simulink model "Stabilize_mode_discretized"  (R2016a)
settings: Solver=VariableStepAuto  StartTime=0.0  StopTime=10  FixedStep=0.0000001  RelTol=1e-3
model workspace (MAT data in the model file):
  AC_ATTITUDE_ACCEL_Y_CONTROLLER_MAX_RADSS = Simulink.Signal
  AC_ATTITUDE_ACCEL_Y_CONTROLLER_MAX_RADSS.DataType = 'double'
  AC_ATTITUDE_ACCEL_Y_CONTROLLER_MAX_RADSS.Dimensions = 1
  AC_ATTITUDE_ACCEL_Y_CONTROLLER_MAX_RADSS.DimensionsMode = 'auto'
  AC_ATTITUDE_ACCEL_Y_CONTROLLER_MAX_RADSS.Complexity = 'real'
  AC_ATTITUDE_ACCEL_Y_CONTROLLER_MAX_RADSS.SampleTime = -1
  AC_ATTITUDE_ACCEL_Y_CONTROLLER_MAX_RADSS.SamplingMode = 'Sample based'
  AC_ATTITUDE_ACCEL_Y_CONTROLLER_MAX_RADSS.InitialValue = '0.5'
  AC_ATTITUDE_CONTROL_MAX = Simulink.Signal
  AC_ATTITUDE_CONTROL_MAX.DataType = 'double'
  AC_ATTITUDE_CONTROL_MAX.Dimensions = 1
  AC_ATTITUDE_CONTROL_MAX.DimensionsMode = 'auto'
  AC_ATTITUDE_CONTROL_MAX.Complexity = 'real'
  AC_ATTITUDE_CONTROL_MAX.SampleTime = -1
  AC_ATTITUDE_CONTROL_MAX.SamplingMode = 'Sample based'
  AC_ATTITUDE_CONTROL_MAX.InitialValue = '0.5'
  AC_ATTITUDE_THRUST_ERROR_ANGLE = Simulink.Signal
  AC_ATTITUDE_THRUST_ERROR_ANGLE.DataType = 'double'
  AC_ATTITUDE_THRUST_ERROR_ANGLE.Dimensions = 1
  AC_ATTITUDE_THRUST_ERROR_ANGLE.DimensionsMode = 'auto'
  AC_ATTITUDE_THRUST_ERROR_ANGLE.Complexity = 'real'
  AC_ATTITUDE_THRUST_ERROR_ANGLE.SampleTime = -1
  AC_ATTITUDE_THRUST_ERROR_ANGLE.SamplingMode = 'Sample based'
  AC_ATTITUDE_THRUST_ERROR_ANGLE.InitialValue = '1000'
  ROLL_PITCH_INPUT_MAX = Simulink.Signal
  ROLL_PITCH_INPUT_MAX.DataType = 'double'
  ROLL_PITCH_INPUT_MAX.Dimensions = 1
  ROLL_PITCH_INPUT_MAX.DimensionsMode = 'auto'
  ROLL_PITCH_INPUT_MAX.Complexity = 'real'
  ROLL_PITCH_INPUT_MAX.SampleTime = -1
  ROLL_PITCH_INPUT_MAX.SamplingMode = 'Sample based'
  ROLL_PITCH_INPUT_MAX.InitialValue = '3000'
  Sig = Simulink.Signal
  Sig.DataType = 'auto'
  Sig.Dimensions = -1
  Sig.DimensionsMode = 'auto'
  Sig.Complexity = 'auto'
  Sig.SampleTime = -1
  Sig.SamplingMode = 'auto'
  Sig1 = Simulink.Signal
  Sig1.DataType = 'auto'
  Sig1.Dimensions = -1
  Sig1.DimensionsMode = 'auto'
  Sig1.Complexity = 'auto'
  Sig1.SampleTime = -1
  Sig1.SamplingMode = 'auto'
  acro_yaw_p = Simulink.Signal
  acro_yaw_p.DataType = 'double'
  acro_yaw_p.Dimensions = 1
  acro_yaw_p.DimensionsMode = 'auto'
  acro_yaw_p.Complexity = 'real'
  acro_yaw_p.SampleTime = -1
  acro_yaw_p.SamplingMode = 'Sample based'
  acro_yaw_p.InitialValue = '45'
  angle_max = Simulink.Signal
  angle_max.DataType = 'double'
  angle_max.Dimensions = 1
  angle_max.DimensionsMode = 'auto'
  angle_max.Complexity = 'real'
  angle_max.SampleTime = -1
  angle_max.SamplingMode = 'Sample based'
  angle_max.InitialValue = '3000'
  attitude_target_ang_vel = Simulink.Signal
  attitude_target_ang_vel.DataType = 'double'
  attitude_target_ang_vel.Dimensions = 3
  attitude_target_ang_vel.DimensionsMode = 'auto'
  attitude_target_ang_vel.Complexity = 'real'
  attitude_target_ang_vel.SampleTime = -1
  attitude_target_ang_vel.SamplingMode = 'Sample based'
  attitude_target_ang_vel.InitialValue = '[0 0 0]'
  attitude_target_euler_angle_x = Simulink.Signal
  attitude_target_euler_angle_x.DataType = 'double'
  attitude_target_euler_angle_x.Dimensions = 1
  attitude_target_euler_angle_x.DimensionsMode = 'auto'
  attitude_target_euler_angle_x.Complexity = 'real'
  attitude_target_euler_angle_x.SampleTime = -1
  attitude_target_euler_angle_x.SamplingMode = 'Sample based'
  attitude_target_euler_angle_x.InitialValue = '0'
  attitude_target_euler_angle_y = Simulink.Signal
  attitude_target_euler_angle_y.DataType = 'double'
  attitude_target_euler_angle_y.Dimensions = 1
  attitude_target_euler_angle_y.DimensionsMode = 'auto'
  attitude_target_euler_angle_y.Complexity = 'real'
  attitude_target_euler_angle_y.SampleTime = -1
  attitude_target_euler_angle_y.SamplingMode = 'Sample based'
  attitude_target_euler_angle_y.InitialValue = '0'
  attitude_target_euler_angle_z = Simulink.Signal
  attitude_target_euler_angle_z.DataType = 'double'
  attitude_target_euler_angle_z.Dimensions = 1
  attitude_target_euler_angle_z.DimensionsMode = 'auto'
  attitude_target_euler_angle_z.Complexity = 'real'
  attitude_target_euler_angle_z.SampleTime = -1
  attitude_target_euler_angle_z.SamplingMode = 'Sample based'
  attitude_target_euler_angle_z.InitialValue = '0'
  attitude_target_euler_rate = Simulink.Signal
  attitude_target_euler_rate.DataType = 'double'
  attitude_target_euler_rate.Dimensions = 3
  attitude_target_euler_rate.DimensionsMode = 'auto'
  attitude_target_euler_rate.Complexity = 'real'
  attitude_target_euler_rate.SampleTime = -1
  attitude_target_euler_rate.SamplingMode = 'Sample based'
  attitude_target_euler_rate.InitialValue = '[0 0 0]'
  attitude_target_quat = Simulink.Signal
  attitude_target_quat.DataType = 'double'
  attitude_target_quat.Dimensions = 4
  attitude_target_quat.DimensionsMode = 'auto'
  attitude_target_quat.Complexity = 'real'
  attitude_target_quat.SampleTime = -1
  attitude_target_quat.SamplingMode = 'Sample based'
  attitude_target_quat.InitialValue = '[1 0 0 0]'
  attitude_vehicle_quat = Simulink.Signal
  attitude_vehicle_quat.DataType = 'double'
  attitude_vehicle_quat.Dimensions = 4
  attitude_vehicle_quat.DimensionsMode = 'auto'
  attitude_vehicle_quat.Complexity = 'real'
  attitude_vehicle_quat.SampleTime = -1
  attitude_vehicle_quat.SamplingMode = 'Sample based'
  attitude_vehicle_quat.InitialValue = '[1 0 0 0]'
  dt = Simulink.Signal
  dt.DataType = 'double'
  dt.Dimensions = 1
  dt.DimensionsMode = 'auto'
  dt.Complexity = 'real'
  dt.SampleTime = -1
  dt.SamplingMode = 'Sample based'
  dt.InitialValue = '0.01'
  false = 0
  limit_roll_pitch = Simulink.Signal
  limit_roll_pitch.DataType = 'double'
  limit_roll_pitch.Dimensions = 1
  limit_roll_pitch.DimensionsMode = 'auto'
  limit_roll_pitch.Complexity = 'real'
  limit_roll_pitch.SampleTime = -1
  limit_roll_pitch.SamplingMode = 'Sample based'
  limit_roll_pitch.InitialValue = '0.0'
  limit_throttle_upper = Simulink.Signal
  limit_throttle_upper.DataType = 'logical'
  limit_throttle_upper.Dimensions = 1
  limit_throttle_upper.DimensionsMode = 'auto'
  limit_throttle_upper.Complexity = 'real'
  limit_throttle_upper.SampleTime = -1
  limit_throttle_upper.SamplingMode = 'Sample based'
  limit_throttle_upper.InitialValue = '0'
  limit_yaw = Simulink.Signal
  limit_yaw.DataType = 'double'
  limit_yaw.Dimensions = 1
  limit_yaw.DimensionsMode = 'auto'
  limit_yaw.Complexity = 'real'
  limit_yaw.SampleTime = -1
  limit_yaw.SamplingMode = 'Sample based'
  limit_yaw.InitialValue = '0'
  loop_rate = Simulink.Signal
  loop_rate.DataType = 'double'
  loop_rate.Dimensions = 1
  loop_rate.DimensionsMode = 'auto'
  loop_rate.Complexity = 'real'
  loop_rate.SampleTime = -1
  loop_rate.SamplingMode = 'Sample based'
  loop_rate.InitialValue = '100'
  pitch_attitude_kP = Simulink.Signal
  pitch_attitude_kP.DataType = 'double'
  pitch_attitude_kP.Dimensions = 1
  pitch_attitude_kP.DimensionsMode = 'auto'
  pitch_attitude_kP.Complexity = 'real'
  pitch_attitude_kP.SampleTime = -1
  pitch_attitude_kP.SamplingMode = 'Sample based'
  pitch_attitude_kP.InitialValue = '20'
  pitch_factor = Simulink.Signal
  pitch_factor.DataType = 'double'
  pitch_factor.Dimensions = 4
  pitch_factor.DimensionsMode = 'auto'
  pitch_factor.Complexity = 'real'
  pitch_factor.SampleTime = -1
  pitch_factor.SamplingMode = 'Sample based'
  pitch_factor.InitialValue = '[cos(deg2rad(15)) -cos(deg2rad(15)) cos(deg2rad(15)) -cos(deg2rad(15))]'
  pitch_rate_derivative = Simulink.Signal
  pitch_rate_derivative.DataType = 'double'
  pitch_rate_derivative.Dimensions = 1
  pitch_rate_derivative.DimensionsMode = 'auto'
  pitch_rate_derivative.Complexity = 'real'
  pitch_rate_derivative.SampleTime = -1
  pitch_rate_derivative.SamplingMode = 'Sample based'
  pitch_rate_derivative.InitialValue = '0'
  pitch_rate_error_rads = Simulink.Signal
  pitch_rate_error_rads.DataType = 'double'
  pitch_rate_error_rads.Dimensions = 1
  pitch_rate_error_rads.DimensionsMode = 'auto'
  pitch_rate_error_rads.Complexity = 'real'
  pitch_rate_error_rads.SampleTime = -1
  pitch_rate_error_rads.SamplingMode = 'Sample based'
  pitch_rate_error_rads.InitialValue = '0'
  pitch_rate_filt_hz = Simulink.Signal
  pitch_rate_filt_hz.DataType = 'double'
  pitch_rate_filt_hz.Dimensions = 1
  pitch_rate_filt_hz.DimensionsMode = 'auto'
  pitch_rate_filt_hz.Complexity = 'real'
  pitch_rate_filt_hz.SampleTime = -1
  pitch_rate_filt_hz.SamplingMode = 'Sample based'
  pitch_rate_filt_hz.InitialValue = '1/(2*pi)'
  pitch_rate_imax = Simulink.Signal
  pitch_rate_imax.DataType = 'double'
  pitch_rate_imax.Dimensions = 1
  pitch_rate_imax.DimensionsMode = 'auto'
  pitch_rate_imax.Complexity = 'real'
  pitch_rate_imax.SampleTime = -1
  pitch_rate_imax.SamplingMode = 'Sample based'
  pitch_rate_imax.InitialValue = '200'
  pitch_rate_integrator = Simulink.Signal
  pitch_rate_integrator.DataType = 'double'
  pitch_rate_integrator.Dimensions = 1
  pitch_rate_integrator.DimensionsMode = 'auto'
  pitch_rate_integrator.Complexity = 'real'
  pitch_rate_integrator.SampleTime = -1
  pitch_rate_integrator.SamplingMode = 'Sample based'
  pitch_rate_integrator.InitialValue = '0'
  pitch_rate_kD = Simulink.Signal
  pitch_rate_kD.DataType = 'double'
  pitch_rate_kD.Dimensions = 1
  pitch_rate_kD.DimensionsMode = 'auto'
  pitch_rate_kD.Complexity = 'real'
  pitch_rate_kD.SampleTime = -1
  pitch_rate_kD.SamplingMode = 'Sample based'
  pitch_rate_kD.InitialValue = '0.004'
  pitch_rate_kI = Simulink.Signal
  pitch_rate_kI.DataType = 'double'
  pitch_rate_kI.Dimensions = 1
  pitch_rate_kI.DimensionsMode = 'auto'
  pitch_rate_kI.Complexity = 'real'
  pitch_rate_kI.SampleTime = -1
  pitch_rate_kI.SamplingMode = 'Sample based'
  pitch_rate_kI.InitialValue = '0.1'
  pitch_rate_kP = Simulink.Signal
  pitch_rate_kP.DataType = 'double'
  pitch_rate_kP.Dimensions = 1
  pitch_rate_kP.DimensionsMode = 'auto'
  pitch_rate_kP.Complexity = 'real'
  pitch_rate_kP.SampleTime = -1
  pitch_rate_kP.SamplingMode = 'Sample based'
  pitch_rate_kP.InitialValue = '0.5'
  pitch_rate_last_input = Simulink.Signal
  pitch_rate_last_input.DataType = 'double'
  pitch_rate_last_input.Dimensions = 1
  pitch_rate_last_input.DimensionsMode = 'auto'
  pitch_rate_last_input.Complexity = 'real'
  pitch_rate_last_input.SampleTime = -1
  pitch_rate_last_input.SamplingMode = 'Sample based'
  pitch_rate_last_input.InitialValue = '0'
  pitch_rate_proportional = Simulink.Signal
  pitch_rate_proportional.DataType = 'double'
  pitch_rate_proportional.Dimensions = 1
  pitch_rate_proportional.DimensionsMode = 'auto'
  pitch_rate_proportional.Complexity = 'real'
  pitch_rate_proportional.SampleTime = -1
  pitch_rate_proportional.SamplingMode = 'Sample based'
  pitch_rate_proportional.InitialValue = '0'
  pwm_max = Simulink.Signal
  pwm_max.DataType = 'double'
  pwm_max.Dimensions = 1
  pwm_max.DimensionsMode = 'auto'
  pwm_max.Complexity = 'real'
  pwm_max.SampleTime = -1
  pwm_max.SamplingMode = 'Sample based'
  pwm_max.InitialValue = '2000'
  pwm_min = Simulink.Signal
  pwm_min.DataType = 'double'
  pwm_min.Dimensions = 1
  pwm_min.DimensionsMode = 'auto'
  pwm_min.Complexity = 'real'
  pwm_min.SampleTime = -1
  pwm_min.SamplingMode = 'Sample based'
  pwm_min.InitialValue = '1039'
  rate_bf_ff_enabled = Simulink.Signal
  rate_bf_ff_enabled.DataType = 'double'
  rate_bf_ff_enabled.Dimensions = 1
  rate_bf_ff_enabled.DimensionsMode = 'auto'
  rate_bf_ff_enabled.Complexity = 'real'
  rate_bf_ff_enabled.SampleTime = -1
  rate_bf_ff_enabled.SamplingMode = 'Sample based'
  rate_bf_ff_enabled.InitialValue = '0'
  rate_target_ang_vel = Simulink.Signal
  rate_target_ang_vel.DataType = 'double'
  rate_target_ang_vel.Dimensions = 3
  rate_target_ang_vel.DimensionsMode = 'auto'
  rate_target_ang_vel.Complexity = 'real'
  rate_target_ang_vel.SampleTime = -1
  rate_target_ang_vel.SamplingMode = 'Sample based'
  rate_target_ang_vel.InitialValue = '[0 0 0]'
  roll_attitude_kP = Simulink.Signal
  roll_attitude_kP.DataType = 'double'
  roll_attitude_kP.Dimensions = 1
  roll_attitude_kP.DimensionsMode = 'auto'
  roll_attitude_kP.Complexity = 'real'
  roll_attitude_kP.SampleTime = -1
  roll_attitude_kP.SamplingMode = 'Sample based'
  roll_attitude_kP.InitialValue = '20'
  roll_factor = Simulink.Signal
  roll_factor.DataType = 'double'
  roll_factor.Dimensions = 4
  roll_factor.DimensionsMode = 'auto'
  roll_factor.Complexity = 'real'
  roll_factor.SampleTime = -1
  roll_factor.SamplingMode = 'Sample based'
  roll_factor.InitialValue = '[-sin(deg2rad(15)) sin(deg2rad(15)) sin(deg2rad(15)) -sin(deg2rad(15))]'
  roll_rate_derivative = Simulink.Signal
  roll_rate_derivative.DataType = 'double'
  roll_rate_derivative.Dimensions = 1
  roll_rate_derivative.DimensionsMode = 'auto'
  roll_rate_derivative.Complexity = 'real'
  roll_rate_derivative.SampleTime = -1
  roll_rate_derivative.SamplingMode = 'Sample based'
  roll_rate_derivative.InitialValue = '0'
  roll_rate_error_rads = Simulink.Signal
  roll_rate_error_rads.DataType = 'double'
  roll_rate_error_rads.Dimensions = 1
  roll_rate_error_rads.DimensionsMode = 'auto'
  roll_rate_error_rads.Complexity = 'real'
  roll_rate_error_rads.SampleTime = -1
  roll_rate_error_rads.SamplingMode = 'Sample based'
  roll_rate_error_rads.InitialValue = '0'
  roll_rate_filt_hz = Simulink.Signal
  roll_rate_filt_hz.DataType = 'double'
  roll_rate_filt_hz.Dimensions = 1
  roll_rate_filt_hz.DimensionsMode = 'auto'
  roll_rate_filt_hz.Complexity = 'real'
  roll_rate_filt_hz.SampleTime = -1
  roll_rate_filt_hz.SamplingMode = 'Sample based'
  roll_rate_filt_hz.InitialValue = '1/(2*pi)'
  roll_rate_imax = Simulink.Signal
  roll_rate_imax.DataType = 'double'
  roll_rate_imax.Dimensions = 1
  roll_rate_imax.DimensionsMode = 'auto'
  roll_rate_imax.Complexity = 'real'
  roll_rate_imax.SampleTime = -1
  roll_rate_imax.SamplingMode = 'Sample based'
  roll_rate_imax.InitialValue = '200'
  roll_rate_integrator = Simulink.Signal
  roll_rate_integrator.DataType = 'double'
  roll_rate_integrator.Dimensions = 1
  roll_rate_integrator.DimensionsMode = 'auto'
  roll_rate_integrator.Complexity = 'real'
  roll_rate_integrator.SampleTime = -1
  roll_rate_integrator.SamplingMode = 'Sample based'
  roll_rate_integrator.InitialValue = '0'
  roll_rate_kD = Simulink.Signal
  roll_rate_kD.DataType = 'double'
  roll_rate_kD.Dimensions = 1
  roll_rate_kD.DimensionsMode = 'auto'
  roll_rate_kD.Complexity = 'real'
  roll_rate_kD.SampleTime = -1
  roll_rate_kD.SamplingMode = 'Sample based'
  roll_rate_kD.InitialValue = '0.004'
  roll_rate_kI = Simulink.Signal
  roll_rate_kI.DataType = 'double'
  roll_rate_kI.Dimensions = 1
  roll_rate_kI.DimensionsMode = 'auto'
  roll_rate_kI.Complexity = 'real'
  roll_rate_kI.SampleTime = -1
  roll_rate_kI.SamplingMode = 'Sample based'
  roll_rate_kI.InitialValue = '0.1'
  roll_rate_kP = Simulink.Signal
  roll_rate_kP.DataType = 'double'
  roll_rate_kP.Dimensions = 1
  roll_rate_kP.DimensionsMode = 'auto'
  roll_rate_kP.Complexity = 'real'
  roll_rate_kP.SampleTime = -1
  roll_rate_kP.SamplingMode = 'Sample based'
  roll_rate_kP.InitialValue = '1'
  roll_rate_last_input = Simulink.Signal
  roll_rate_last_input.DataType = 'double'
  roll_rate_last_input.Dimensions = 1
  roll_rate_last_input.DimensionsMode = 'auto'
  roll_rate_last_input.Complexity = 'real'
  roll_rate_last_input.SampleTime = -1
  roll_rate_last_input.SamplingMode = 'Sample based'
  roll_rate_last_input.InitialValue = '0'
  roll_rate_proportional = Simulink.Signal
  roll_rate_proportional.DataType = 'double'
  roll_rate_proportional.Dimensions = 1
  roll_rate_proportional.DimensionsMode = 'auto'
  roll_rate_proportional.Complexity = 'real'
  roll_rate_proportional.SampleTime = -1
  roll_rate_proportional.SamplingMode = 'Sample based'
  roll_rate_proportional.InitialValue = '0'
  spin_max = Simulink.Signal
  spin_max.DataType = 'double'
  spin_max.Dimensions = 1
  spin_max.DimensionsMode = 'auto'
  spin_max.Complexity = 'real'
  spin_max.SampleTime = -1
  spin_max.SamplingMode = 'Sample based'
  spin_max.InitialValue = '0.95'
  spin_min = Simulink.Signal
  spin_min.DataType = 'double'
  spin_min.Dimensions = 1
  spin_min.DimensionsMode = 'auto'
  spin_min.Complexity = 'real'
  spin_min.SampleTime = -1
  spin_min.SamplingMode = 'Sample based'
  spin_min.InitialValue = '0.15'
  throttle_avg_max = Simulink.Signal
  throttle_avg_max.DataType = 'double'
  throttle_avg_max.Dimensions = 1
  throttle_avg_max.DimensionsMode = 'auto'
  throttle_avg_max.Complexity = 'real'
  throttle_avg_max.SampleTime = -1
  throttle_avg_max.SamplingMode = 'Sample based'
  throttle_avg_max.InitialValue = '0'
  throttle_filter_cutoff_freq = Simulink.Signal
  throttle_filter_cutoff_freq.DataType = 'double'
  throttle_filter_cutoff_freq.Dimensions = 1
  throttle_filter_cutoff_freq.DimensionsMode = 'auto'
  throttle_filter_cutoff_freq.Complexity = 'real'
  throttle_filter_cutoff_freq.SampleTime = -1
  throttle_filter_cutoff_freq.SamplingMode = 'Sample based'
  throttle_filter_cutoff_freq.InitialValue = '0.5'
  throttle_filter_output = Simulink.Signal
  throttle_filter_output.DataType = 'double'
  throttle_filter_output.Dimensions = 1
  throttle_filter_output.DimensionsMode = 'auto'
  throttle_filter_output.Complexity = 'real'
  throttle_filter_output.SampleTime = -1
  throttle_filter_output.SamplingMode = 'Sample based'
  throttle_filter_output.InitialValue = '0'
  throttle_in = Simulink.Signal
  throttle_in.DataType = 'double'
  throttle_in.Dimensions = 1
  throttle_in.DimensionsMode = 'auto'
  throttle_in.Complexity = 'real'
  throttle_in.SampleTime = -1
  throttle_in.SamplingMode = 'Sample based'
  throttle_in.InitialValue = '0'
  throttle_rpy_mix = Simulink.Signal
  throttle_rpy_mix.DataType = 'double'
  throttle_rpy_mix.Dimensions = 1
  throttle_rpy_mix.DimensionsMode = 'auto'
  throttle_rpy_mix.Complexity = 'real'
  throttle_rpy_mix.SampleTime = -1
  throttle_rpy_mix.SamplingMode = 'Sample based'
  throttle_rpy_mix.InitialValue = '0'
  throttle_rpy_mix_desired = Simulink.Signal
  throttle_rpy_mix_desired.DataType = 'double'
  throttle_rpy_mix_desired.Dimensions = 1
  throttle_rpy_mix_desired.DimensionsMode = 'auto'
  throttle_rpy_mix_desired.Complexity = 'real'
  throttle_rpy_mix_desired.SampleTime = -1
  throttle_rpy_mix_desired.SamplingMode = 'Sample based'
  throttle_rpy_mix_desired.InitialValue = '0'
  throttle_thrust = Simulink.Signal
  throttle_thrust.DataType = 'double'
  throttle_thrust.Dimensions = 1
  throttle_thrust.DimensionsMode = 'auto'
  throttle_thrust.Complexity = 'real'
  throttle_thrust.SampleTime = -1
  throttle_thrust.SamplingMode = 'Sample based'
  throttle_thrust.InitialValue = '0'
  throttle_thrust_best_rpy = Simulink.Signal
  throttle_thrust_best_rpy.DataType = 'double'
  throttle_thrust_best_rpy.Dimensions = 1
  throttle_thrust_best_rpy.DimensionsMode = 'auto'
  throttle_thrust_best_rpy.Complexity = 'real'
  throttle_thrust_best_rpy.SampleTime = -1
  throttle_thrust_best_rpy.SamplingMode = 'Sample based'
  throttle_thrust_best_rpy.InitialValue = '0'
  throttle_thrust_max = Simulink.Signal
  throttle_thrust_max.DataType = 'double'
  throttle_thrust_max.Dimensions = 1
  throttle_thrust_max.DimensionsMode = 'auto'
  throttle_thrust_max.Complexity = 'real'
  throttle_thrust_max.SampleTime = -1
  throttle_thrust_max.SamplingMode = 'Sample based'
  throttle_thrust_max.InitialValue = '1'
  thrust_error_angle = Simulink.Signal
  thrust_error_angle.DataType = 'double'
  thrust_error_angle.Dimensions = 1
  thrust_error_angle.DimensionsMode = 'auto'
  thrust_error_angle.Complexity = 'real'
  thrust_error_angle.SampleTime = -1
  thrust_error_angle.SamplingMode = 'Sample based'
  thrust_error_angle.InitialValue = '0'
  thrust_rpyt_out = Simulink.Signal
  thrust_rpyt_out.DataType = 'double'
  thrust_rpyt_out.Dimensions = 4
  thrust_rpyt_out.DimensionsMode = 'auto'
  thrust_rpyt_out.Complexity = 'real'
  thrust_rpyt_out.SampleTime = -1
  thrust_rpyt_out.SamplingMode = 'Sample based'
  thrust_rpyt_out.InitialValue = '[0 0 0 0]'
  true = 1
  use_ff_and_input_shaping = Simulink.Signal
  use_ff_and_input_shaping.DataType = 'double'
  use_ff_and_input_shaping.Dimensions = 1
  use_ff_and_input_shaping.DimensionsMode = 'auto'
  use_ff_and_input_shaping.Complexity = 'real'
  use_ff_and_input_shaping.SampleTime = -1
  use_ff_and_input_shaping.SamplingMode = 'Sample based'
  use_ff_and_input_shaping.InitialValue = '0'
  variableType = 'S'
  yaw_allowed = Simulink.Signal
  yaw_allowed.DataType = 'double'
  yaw_allowed.Dimensions = 1
  yaw_allowed.DimensionsMode = 'auto'
  yaw_allowed.Complexity = 'real'
  yaw_allowed.SampleTime = -1
  yaw_allowed.SamplingMode = 'Sample based'
  yaw_allowed.InitialValue = '1'
  yaw_attitude_kP = Simulink.Signal
  yaw_attitude_kP.DataType = 'double'
  yaw_attitude_kP.Dimensions = 1
  yaw_attitude_kP.DimensionsMode = 'auto'
  yaw_attitude_kP.Complexity = 'real'
  yaw_attitude_kP.SampleTime = -1
  yaw_attitude_kP.SamplingMode = 'Sample based'
  yaw_attitude_kP.InitialValue = '4.5'
  yaw_factor = Simulink.Signal
  yaw_factor.DataType = 'double'
  yaw_factor.Dimensions = 4
  yaw_factor.DimensionsMode = 'auto'
  yaw_factor.Complexity = 'real'
  yaw_factor.SampleTime = -1
  yaw_factor.SamplingMode = 'Sample based'
  yaw_factor.InitialValue = '[0.1 0.1 -0.1 -0.1]'
  yaw_headroom = Simulink.Signal
  yaw_headroom.DataType = 'double'
  yaw_headroom.Dimensions = 1
  yaw_headroom.DimensionsMode = 'auto'
  yaw_headroom.Complexity = 'real'
  yaw_headroom.SampleTime = -1
  yaw_headroom.SamplingMode = 'Sample based'
  yaw_headroom.InitialValue = '200'
  yaw_rate_derivative = Simulink.Signal
  yaw_rate_derivative.DataType = 'double'
  yaw_rate_derivative.Dimensions = 1
  yaw_rate_derivative.DimensionsMode = 'auto'
  yaw_rate_derivative.Complexity = 'real'
  yaw_rate_derivative.SampleTime = -1
  yaw_rate_derivative.SamplingMode = 'Sample based'
  yaw_rate_derivative.InitialValue = '0'
  yaw_rate_error_rads = Simulink.Signal
  yaw_rate_error_rads.DataType = 'double'
  yaw_rate_error_rads.Dimensions = 1
  yaw_rate_error_rads.DimensionsMode = 'auto'
  yaw_rate_error_rads.Complexity = 'real'
  yaw_rate_error_rads.SampleTime = -1
  yaw_rate_error_rads.SamplingMode = 'Sample based'
  yaw_rate_error_rads.InitialValue = '0'
  yaw_rate_filt_hz = Simulink.Signal
  yaw_rate_filt_hz.DataType = 'double'
  yaw_rate_filt_hz.Dimensions = 1
  yaw_rate_filt_hz.DimensionsMode = 'auto'
  yaw_rate_filt_hz.Complexity = 'real'
  yaw_rate_filt_hz.SampleTime = -1
  yaw_rate_filt_hz.SamplingMode = 'Sample based'
  yaw_rate_filt_hz.InitialValue = '1/(2*pi)'
  yaw_rate_imax = Simulink.Signal
  yaw_rate_imax.DataType = 'double'
  yaw_rate_imax.Dimensions = 1
  yaw_rate_imax.DimensionsMode = 'auto'
  yaw_rate_imax.Complexity = 'real'
  yaw_rate_imax.SampleTime = -1
  yaw_rate_imax.SamplingMode = 'Sample based'
  yaw_rate_imax.InitialValue = '200'
  yaw_rate_integrator = Simulink.Signal
  yaw_rate_integrator.DataType = 'double'
  yaw_rate_integrator.Dimensions = 1
  yaw_rate_integrator.DimensionsMode = 'auto'
  yaw_rate_integrator.Complexity = 'real'
  yaw_rate_integrator.SampleTime = -1
  yaw_rate_integrator.SamplingMode = 'Sample based'
  yaw_rate_integrator.InitialValue = '0'
  yaw_rate_kD = Simulink.Signal
  yaw_rate_kD.DataType = 'double'
  yaw_rate_kD.Dimensions = 1
  yaw_rate_kD.DimensionsMode = 'auto'
  yaw_rate_kD.Complexity = 'real'
  yaw_rate_kD.SampleTime = -1
  yaw_rate_kD.SamplingMode = 'Sample based'
  yaw_rate_kD.InitialValue = '5'
  yaw_rate_kI = Simulink.Signal
  yaw_rate_kI.DataType = 'double'
  yaw_rate_kI.Dimensions = 1
  yaw_rate_kI.DimensionsMode = 'auto'
  yaw_rate_kI.Complexity = 'real'
  yaw_rate_kI.SampleTime = -1
  yaw_rate_kI.SamplingMode = 'Sample based'
  yaw_rate_kI.InitialValue = '0.1'
  yaw_rate_kP = Simulink.Signal
  yaw_rate_kP.DataType = 'double'
  yaw_rate_kP.Dimensions = 1
  yaw_rate_kP.DimensionsMode = 'auto'
  yaw_rate_kP.Complexity = 'real'
  yaw_rate_kP.SampleTime = -1
  yaw_rate_kP.SamplingMode = 'Sample based'
  yaw_rate_kP.InitialValue = '0.2'
  yaw_rate_last_input = Simulink.Signal
  yaw_rate_last_input.DataType = 'double'
  yaw_rate_last_input.Dimensions = 1
  yaw_rate_last_input.DimensionsMode = 'auto'
  yaw_rate_last_input.Complexity = 'real'
  yaw_rate_last_input.SampleTime = -1
  yaw_rate_last_input.SamplingMode = 'Sample based'
  yaw_rate_last_input.InitialValue = '0'
  yaw_rate_proportional = Simulink.Signal
  yaw_rate_proportional.DataType = 'double'
  yaw_rate_proportional.Dimensions = 1
  yaw_rate_proportional.DimensionsMode = 'auto'
  yaw_rate_proportional.Complexity = 'real'
  yaw_rate_proportional.SampleTime = -1
  yaw_rate_proportional.SamplingMode = 'Sample based'
  yaw_rate_proportional.InitialValue = '0'
values from neighbouring files (symbols this model uses):
  A = [0 0  0 1 0 0 0 0 0 0 0 0 ... (first row only)    [attitudeMatrices.m]
  B = [0   0   0    0    0    0 ... (first row only)    [attitudeMatrices.m]
  C = [1 0 0 0 0 0 0 0 0 0 0 0 ... (first row only)    [attitudeMatrices.m]
  D = zeros(12,6)    [attitudeMatrices.m]
  Ix = 0.026    [attitudeMatrices.m]
  Iy = 0.15    [attitudeMatrices.m]
  Iz = 0.18    [attitudeMatrices.m]
  R = diag([QR1(2) QR2(2) QR3(2) QR4(2) QR5(2) QR6(2) QR7(2) QR8(2) QR9(2) QR10(2) QR11(2) QR12(2)])    [attitudeMatrices.m]
undefined symbols (not defined in the file or in its folder): Discrete, dtzoh, Time, Ts
libraries: aerolibactuator x2, simulink x2, aerolib6dof2 x1, ctrlSharedLib x1, aerolibconvert2 x1
settings Model: Creator=s121814  LastModifiedBy=GusBus
settings SolverCC: ZeroCrossControl=DisableAll
settings DataIOCC: SaveFormat=Array  SaveState=on

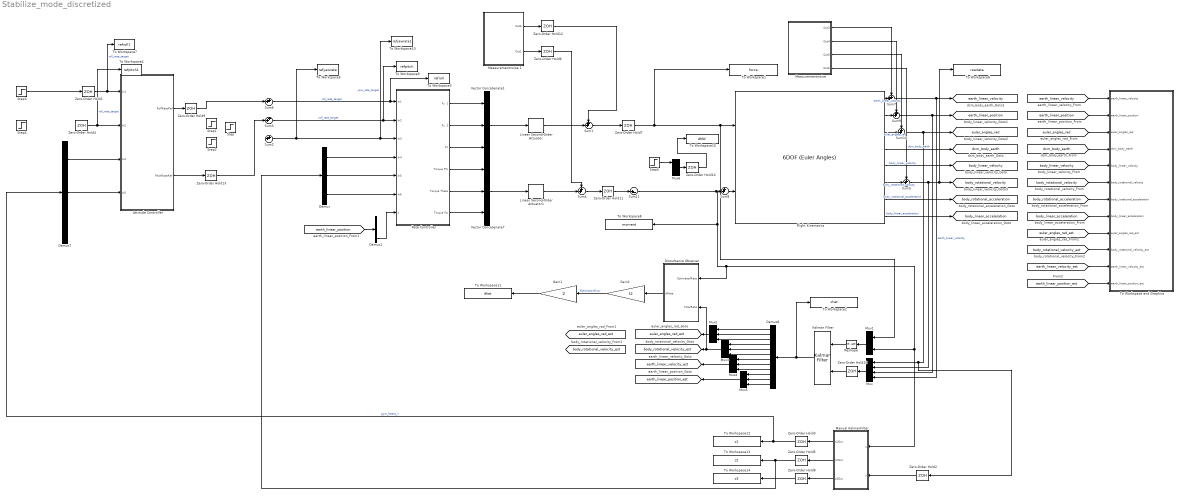
== system Stabilize_mode_discretized ==
  Attitude Controller : Subsystem
  Demux : Demux  Outputs=3
  Demux1 : Demux  Outputs=3
  Demux6 : Demux  Outputs=12
  Demux7 : Demux  Outputs=3
  Disturbance Observer : Subsystem
  Flight Kinematics : aerolib6dof2/6DOF (Euler Angles)  units=Metric (MKS)  mtype=Fixed  rep=Euler Angles  xme_0=[0 0 0]  Vm_0=[0 0 0]  eul_0=[0 0 0]  pm_0=[0 0 0]  mass_0=3.352  mass_e=0.5  mass_f=2.0  inertia=[0.025028 0 0; 0 0.16926 0; 0 0 0.170197]  inertia_e=eye(3)  inertia_f=2*eye(3)  k_quat=1.0  vre_flag=on
  Gain1 : Gain  Gain=2
  Gain2 : Gain  Gain=Iz
  Kalman Filter : ctrlSharedLib/Kalman Filter  TimeDomain=Discrete-Time  UseCurrentEstimator=on  ModelSource=Individual A, B, C, D matrices  ModelSourceVariable=ss(0.95,1,1,0,1)  A=A  B=B  C=C  D=D  NumberOfStates=1  NumberOfInputs=1  NumberOfOutputs=1  InitialEstimateSource=Dialog  X0=zeros(12,1)  P0=10  UseK=off  UseGH=off  NumberOfProcessNoiseInputs=1  G=1  TimeInvariantG=on  H=0  TimeInvariantH=on  Q=Q  TimeInvariantQ=on  R=R  TimeInvariantR=on  N=0  TimeInvariantN=on  AddInputPort=on  AddEnablePort=off  ExternalReset=none  OutputEstimatedY=off  OutputP=off  Ts=-1
  Linear Second-Order Actuator : aerolibactuator/Linear Second-Order Actuator  wn_fin=500  z_fin=1  fin_act_0=0  fin_act_vel=0
  Linear Second-Order Actuator1 : aerolibactuator/Linear Second-Order Actuator  wn_fin=500  z_fin=1  fin_act_0=0  fin_act_vel=0
  Manual KalmanFilter : Subsystem
  "Measurementnoise " : Subsystem
  Measurementnoise 1 : Subsystem
  Mux : Mux
  Mux1 : Mux  Inputs=2
  Mux{2..6} (5 alike) : Mux  Inputs=3
  Rate Controller : Subsystem
  Reshape : Reshape  OutputDimensionality=Customize  OutputDimensions=[6,1]
  Step{,1..4} (5 alike) : Step  Time=0.5  After=10  SampleTime=0
  Step5 : Step  Time=2  After=1.5  SampleTime=0
  Sum{1..10} (10 alike) : Sum  Inputs=++|
  Sum11 : Sum  Inputs=|+-
  To Workspace and Graphics : Subsystem
  To Workspace1 : ToWorkspace  VariableName=force  SampleTime=-1
  To Workspace10 : ToWorkspace  VariableName=refyawrate1  SampleTime=-1
  To Workspace11 : ToWorkspace  VariableName=dhat  SampleTime=-1
  To Workspace12 : ToWorkspace  VariableName=z1  SampleTime=-1
  To Workspace13 : ToWorkspace  VariableName=z2  SampleTime=-1
  To Workspace14 : ToWorkspace  VariableName=z3  SampleTime=-1
  To Workspace15 : ToWorkspace  VariableName=dNW  SampleTime=-1
  To Workspace2 : ToWorkspace  VariableName=xhat  SampleTime=-1
  To Workspace3 : ToWorkspace  VariableName=refroll  SampleTime=-1
  To Workspace4 : ToWorkspace  VariableName=refpitch1  SampleTime=-1
  To Workspace5 : ToWorkspace  VariableName=refyawrate  SampleTime=-1
  To Workspace6 : ToWorkspace  VariableName=rawdata  SampleTime=-1
  To Workspace7 : ToWorkspace  VariableName=refroll1  SampleTime=-1
  To Workspace8 : ToWorkspace  VariableName=moment  SampleTime=-1
  To Workspace9 : ToWorkspace  VariableName=refpitch  SampleTime=-1
  Vector Concatenate1 : Concatenate  NumInputs=3
  Vector Concatenate7 : Concatenate  NumInputs=3
  Zero-Order Hold{1..13,15} (14 alike) : ZeroOrderHold  SampleTime=dtzoh
  tag scope: body_linear_acceleration=global, body_linear_velocity=global, body_rotational_acceleration=global, body_rotational_velocity=global, body_rotational_velocity_est=global, dcm_body_earth=global, earth_linear_position=global, earth_linear_position_est=global, earth_linear_velocity=global, earth_linear_velocity_est=global, euler_angles_rad=global, euler_angles_rad_est=global
  wires:
  [body_rotational_velocity] -> To Workspace and Graphics/6(body_rotational_velocity)
  [body_linear_acceleration] -> To Workspace and Graphics/8(body_linear_acceleration)
  [body_rotational_acceleration] -> To Workspace and Graphics/7(body_rotational_acceleration)
  [body_linear_velocity] -> To Workspace and Graphics/5(body_linear_velocity)
  [dcm_body_earth] -> To Workspace and Graphics/4(dcm_body_earth)
  [euler_angles_rad] -> To Workspace and Graphics/3(euler_angles_rad)
  [earth_linear_position] -> To Workspace and Graphics/2(earth_linear_position)
  [earth_linear_velocity] -> To Workspace and Graphics/1(earth_linear_velocity)
  Sum7/1 -> [earth_linear_velocity], Mux/4  "earth_linear_velocity"
  Flight Kinematics/7 -> [body_rotational_acceleration]  "body_rotational_acceleration"
  Flight Kinematics/8 -> [body_linear_acceleration]  "body_linear_acceleration"
  Flight Kinematics/4 -> [dcm_body_earth]  "dcm_body_earth"
  Flight Kinematics/5 -> [body_linear_velocity]  "body_linear_velocity"
  Sum10/1 -> Zero-Order Hold2/1, Mux/1, [euler_angles_rad]
  Flight Kinematics/3 -> Sum10/2  "euler_angles_rad"
  Sum9/1 -> [earth_linear_position], Mux/3
  Flight Kinematics/2 -> Sum9/2
  Flight Kinematics/6 -> Sum5/2  "body_rotational_velocity"
  Demux/3 -> Rate Controller/6(In6)
  Demux/2 -> Rate Controller/5(In5)
  Zero-Order Hold3/1 -> Demux7/1, To Workspace12/1  "gyro_latest_x"
  "Measurementnoise "/1(Out3) -> Sum7/1
  "Measurementnoise "/2(Out4) -> Sum9/1
  "Measurementnoise "/3(Out5) -> Sum10/1
  "Measurementnoise "/4(Out6) -> Sum5/1
  Demux1/3 -> Rate Controller/7(z)
  Mux/1 -> Zero-Order Hold15/1
  Demux6/1 -> Mux2/1
  Demux6/2 -> Mux2/2
  Demux6/3 -> Mux2/3
  Demux6/4 -> Mux3/1
  Demux6/5 -> Mux3/2
  Demux6/6 -> Mux3/3
  Demux6/7 -> Mux4/1
  Demux6/8 -> Mux4/2
  Demux6/9 -> Mux4/3
  Demux6/10 -> Mux5/1
  Demux6/11 -> Mux5/2
  Demux6/12 -> Mux5/3
  Measurementnoise 1/1(Out6) -> Zero-Order Hold12/1
  Flight Kinematics/1 -> Sum7/2  "earth_linear_velocity"
  Mux3/1 -> Disturbance Observer/2(TotalRate), [body_rotational_velocity_est]
  Mux2/1 -> [euler_angles_rad_est]
  Mux5/1 -> [earth_linear_position_est]
  Mux4/1 -> [earth_linear_velocity_est]
  [earth_linear_position_est] -> To Workspace and Graphics/12(earth_linear_position_est)
  [earth_linear_velocity_est] -> To Workspace and Graphics/11(earth_linear_velocity_est)
  [body_rotational_velocity_est] -> To Workspace and Graphics/10(body_rotational_velocity_est)
  [euler_angles_rad_est] -> To Workspace and Graphics/9(euler_angles_rad_est)
  Linear Second-Order Actuator1/1 -> Sum4/2
  Linear Second-Order Actuator/1 -> Sum1/2
  Demux7/2 -> Attitude Controller/4(In5)
  Sum2/1 -> Rate Controller/3(In3), To Workspace10/1, To Workspace5/1  "yaw_rate_target"
  [earth_linear_position] -> Demux1/1
  Zero-Order Hold12/1 -> Sum1/1
  Vector Concatenate1/1 -> Linear Second-Order Actuator/1
  Vector Concatenate7/1 -> Linear Second-Order Actuator1/1
  Zero-Order Hold15/1 -> Kalman Filter/2
  Mux1/1 -> Reshape/1
  Kalman Filter/1 -> Demux6/1, To Workspace2/1
  Zero-Order Hold7/1 -> Flight Kinematics/1, Mux1/1, To Workspace1/1
  Measurementnoise 1/2(Out1) -> Zero-Order Hold6/1
  Zero-Order Hold6/1 -> Sum4/1
  Sum5/1 -> Mux/2, To Workspace6/1, [body_rotational_velocity]
  Sum1/1 -> Zero-Order Hold7/1
  Sum4/1 -> Zero-Order Hold11/1
  Sum3/1 -> To Workspace9/1, Rate Controller/2(In2)  "roll_rate_target"
  Disturbance Observer/1(dRate) -> Gain2/1
  Sum8/1 -> Flight Kinematics/2
  Gain2/1 -> Gain1/1  "EstimationError"
  Mux6/1 -> Zero-Order Hold10/1
  Step5/1 -> Mux6/1
  Reshape/1 -> Kalman Filter/1
  Gain1/1 -> To Workspace11/1
  Rate Controller/1(Fz  1) -> Vector Concatenate1/1
  Rate Controller/2(Fz  2) -> Vector Concatenate1/2
  Rate Controller/3("Fz  ") -> Vector Concatenate1/3
  Rate Controller/4(Torque Phi) -> Vector Concatenate7/1
  Rate Controller/5(Torque Theta) -> Vector Concatenate7/2
  Rate Controller/6(Torque Psi) -> Vector Concatenate7/3
  Sum11/1 -> Disturbance Observer/1(EstimatedRate), Manual KalmanFilter/1(u), Mux1/2, To Workspace8/1, Sum8/2
  Zero-Order Hold2/1 -> Manual KalmanFilter/2(y)
  Manual KalmanFilter/1(z1Out) -> Zero-Order Hold3/1
  Manual KalmanFilter/2(z2Out) -> Zero-Order Hold5/1
  Manual KalmanFilter/3(z3Out) -> Zero-Order Hold8/1
  Zero-Order Hold5/1 -> Demux/1, To Workspace13/1
  Zero-Order Hold8/1 -> To Workspace14/1
  Attitude Controller/1(RollRateRef) -> Zero-Order Hold9/1
  Zero-Order Hold1/1 -> To Workspace7/1, Attitude Controller/1(In1)  "roll_rate_target"
  Sum6/1 -> To Workspace3/1, Rate Controller/1(In1)  "roll_rate_target"
  Zero-Order Hold9/1 -> Sum6/2
  Zero-Order Hold10/1 -> To Workspace15/1
  Zero-Order Hold11/1 -> Sum11/1
  Zero-Order Hold4/1 -> To Workspace4/1, Attitude Controller/2(In2)  "roll_rate_target"
  Demux/1 -> Rate Controller/4(In4)
  Demux7/1 -> Attitude Controller/3(In4)
  Attitude Controller/2(PitchRateRef) -> Zero-Order Hold13/1
  Zero-Order Hold13/1 -> Sum3/2
  Step3/1 -> Zero-Order Hold1/1

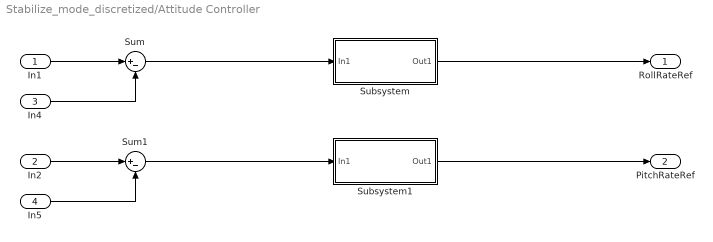
== system Stabilize_mode_discretized/Attitude Controller ==
  In1 : Inport
  In2 : Inport  Port=2
  In4 : Inport  Port=3
  In5 : Inport  Port=4
  Subsystem : Subsystem
  Subsystem1 : Subsystem
  Sum : Sum  Inputs=|+-
  Sum1 : Sum  Inputs=|+-
  RollRateRef : Outport
  PitchRateRef : Outport  Port=2
  wires:
  In1/1 -> Sum/1
  In4/1 -> Sum/2
  In2/1 -> Sum1/1
  In5/1 -> Sum1/2
  Sum/1 -> Subsystem/1(In1)
  Sum1/1 -> Subsystem1/1(In1)
  Subsystem1/1(Out1) -> PitchRateRef/1
  Subsystem/1(Out1) -> RollRateRef/1

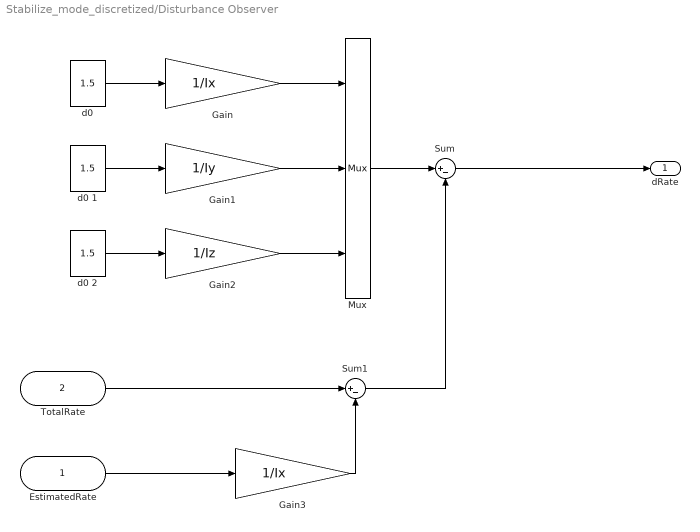
== system Stabilize_mode_discretized/Disturbance Observer ==
  EstimatedRate : Inport
  TotalRate : Inport  Port=2
  Gain : Gain  Gain=1/Ix
  Gain1 : Gain  Gain=1/Iy
  Gain2 : Gain  Gain=1/Iz
  Gain3 : Gain  Gain=1/Ix
  Mux : Mux  Inputs=3
  Sum : Sum  Inputs=|+-
  Sum1 : Sum  Inputs=|+-
  "d0 " : Constant  Value=1.5
  d0 1 : Constant  Value=1.5
  d0 2 : Constant  Value=1.5
  dRate : Outport
  wires:
  "d0 "/1 -> Gain/1
  d0 1/1 -> Gain1/1
  d0 2/1 -> Gain2/1
  Gain/1 -> Mux/1
  Gain1/1 -> Mux/2
  Gain2/1 -> Mux/3
  Mux/1 -> Sum/1
  Sum1/1 -> Sum/2
  TotalRate/1 -> Sum1/1
  Gain3/1 -> Sum1/2
  EstimatedRate/1 -> Gain3/1
  Sum/1 -> dRate/1

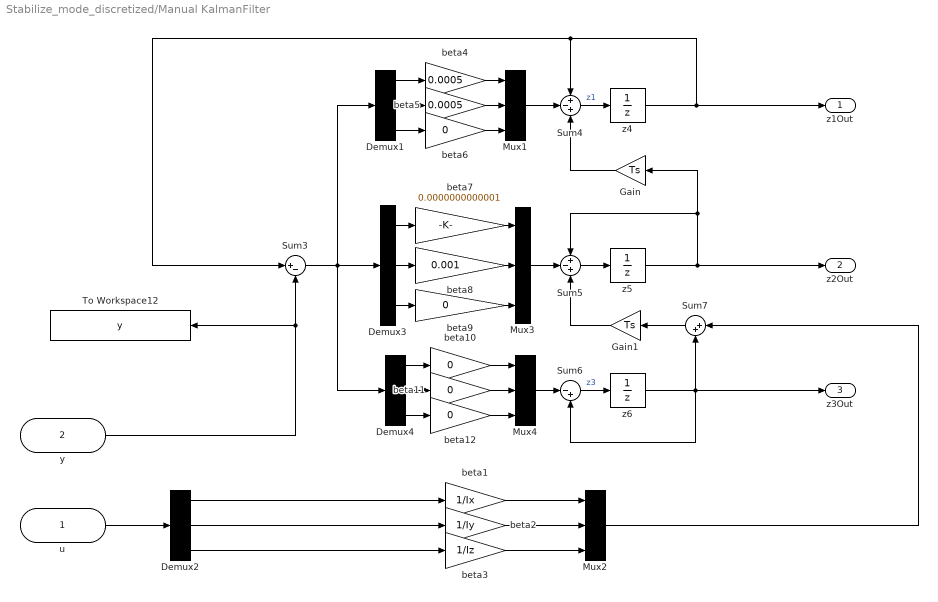
== system Stabilize_mode_discretized/Manual KalmanFilter ==
  u : Inport
  y : Inport  Port=2
  Demux{1..4} (4 alike) : Demux  Outputs=3
  Gain : Gain  Gain=Ts
  Gain1 : Gain  Gain=Ts
  Mux{1..4} (4 alike) : Mux  Inputs=3
  Sum3 : Sum  Inputs=|+-
  Sum4 : Sum  Inputs=+-+
  Sum5 : Sum  Inputs=+-+
  Sum6 : Sum  Inputs=|-+
  Sum7 : Sum  Inputs=|++
  To Workspace12 : ToWorkspace  VariableName=y  SampleTime=-1
  beta1 : Gain  Gain=1/Ix
  beta{6,9..12} (5 alike) : Gain  Gain=0
  beta2 : Gain  Gain=1/Iy
  beta3 : Gain  Gain=1/Iz
  beta4 : Gain  Gain=0.0005
  beta5 : Gain  Gain=0.0005
  beta7 : Gain  Gain=0.0000000000001
  beta8 : Gain  Gain=0.001
  z4 : UnitDelay  SampleTime=Ts
  z5 : UnitDelay  SampleTime=Ts
  z6 : UnitDelay  SampleTime=Ts
  z1Out : Outport
  z2Out : Outport  Port=2
  z3Out : Outport  Port=3
  wires:
  z5/1 -> Gain/1, Sum5/1, z2Out/1
  z4/1 -> Sum3/1, Sum4/1, z1Out/1
  z6/1 -> Sum6/2, Sum7/2, z3Out/1
  Sum3/1 -> Demux1/1, Demux3/1, Demux4/1
  u/1 -> Demux2/1
  Mux1/1 -> Sum4/2
  Sum4/1 -> z4/1  "z1"
  Sum5/1 -> z5/1
  Sum6/1 -> z6/1  "z3"
  Mux4/1 -> Sum6/1
  Sum7/1 -> Gain1/1
  Gain1/1 -> Sum5/3
  Mux3/1 -> Sum5/2
  Gain/1 -> Sum4/3
  Mux2/1 -> Sum7/1
  y/1 -> To Workspace12/1, Sum3/2
  Demux2/1 -> beta1/1
  beta1/1 -> Mux2/1
  Demux2/2 -> beta2/1
  beta2/1 -> Mux2/2
  Demux2/3 -> beta3/1
  beta3/1 -> Mux2/3
  Demux1/1 -> beta4/1
  beta4/1 -> Mux1/1
  Demux1/2 -> beta5/1
  beta5/1 -> Mux1/2
  Demux1/3 -> beta6/1
  beta6/1 -> Mux1/3
  Demux3/1 -> beta7/1
  beta7/1 -> Mux3/1
  Demux3/2 -> beta8/1
  beta8/1 -> Mux3/2
  Demux3/3 -> beta9/1
  beta9/1 -> Mux3/3
  Demux4/1 -> beta10/1
  beta10/1 -> Mux4/1
  Demux4/2 -> beta11/1
  beta11/1 -> Mux4/2
  Demux4/3 -> beta12/1
  beta12/1 -> Mux4/3

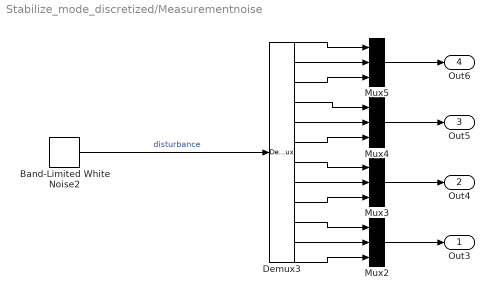
== system Stabilize_mode_discretized/Measurementnoise  ==
  Band-Limited White Noise2 : simulink/Sources/Band-Limited White Noise  Cov=[1 1 1 1 1 1 1 1 1 1 1 1]*0.0001  Ts=0.001  seed=[23341 23341 23341 23341 23341 23341 23341 23341 23341 23341 23341 23341]
  Demux3 : Demux  Outputs=12
  Mux{2..5} (4 alike) : Mux  Inputs=3
  Out3 : Outport
  Out4 : Outport  Port=2
  Out5 : Outport  Port=3
  Out6 : Outport  Port=4
  wires:
  Mux2/1 -> Out3/1
  Demux3/1 -> Mux5/1
  Demux3/9 -> Mux3/3
  Demux3/7 -> Mux3/1
  Demux3/4 -> Mux4/1
  Demux3/5 -> Mux4/2
  Demux3/6 -> Mux4/3
  Demux3/11 -> Mux2/2
  Demux3/2 -> Mux5/2
  Demux3/12 -> Mux2/3
  Demux3/10 -> Mux2/1
  Demux3/3 -> Mux5/3
  Demux3/8 -> Mux3/2
  Mux4/1 -> Out5/1
  Mux5/1 -> Out6/1
  Mux3/1 -> Out4/1
  Band-Limited White Noise2/1 -> Demux3/1  "disturbance"

== system Stabilize_mode_discretized/Measurementnoise 1 ==
  Band-Limited White Noise2 : simulink/Sources/Band-Limited White Noise  Cov=[1 1 1]*0.00001  Ts=0.001  seed=[23341 23341 23341]
  Gain : Gain  Gain=0.1
  Out6 : Outport
  Out1 : Outport  Port=2
  wires:
  Band-Limited White Noise2/1 -> Gain/1, Out6/1  "disturbance"
  Gain/1 -> Out1/1

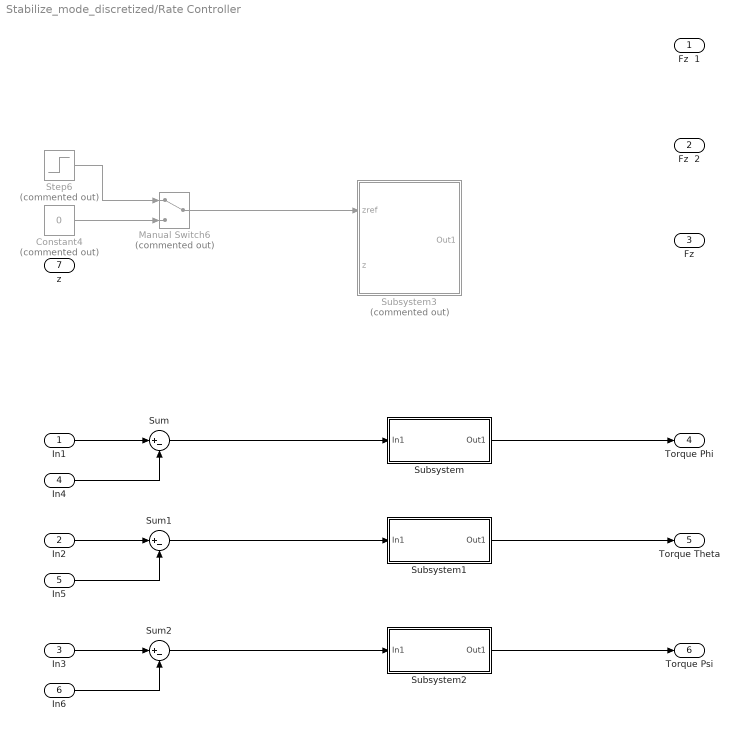
== system Stabilize_mode_discretized/Rate Controller ==
  In1 : Inport
  In2 : Inport  Port=2
  In3 : Inport  Port=3
  In4 : Inport  Port=4
  In5 : Inport  Port=5
  In6 : Inport  Port=6
  z : Inport  Port=7
  Constant4 : Constant  Commented=on  Value=0  SampleTime=0
  Manual Switch6 : ManualSwitch  Commented=on
  Step6 : Step  Commented=on  Time=2  SampleTime=0
  Subsystem : Subsystem
  Subsystem1 : Subsystem
  Subsystem2 : Subsystem
  Subsystem3 : Subsystem  Commented=on
  Sum : Sum  Inputs=|+-
  Sum1 : Sum  Inputs=|+-
  Sum2 : Sum  Inputs=|+-
  Fz  1 : Outport
  Fz  2 : Outport  Port=2
  "Fz  " : Outport  Port=3
  Torque Phi : Outport  Port=4
  Torque Theta : Outport  Port=5
  Torque Psi : Outport  Port=6
  wires:
  In1/1 -> Sum/1
  In4/1 -> Sum/2
  In2/1 -> Sum1/1
  In5/1 -> Sum1/2
  In3/1 -> Sum2/1
  In6/1 -> Sum2/2
  Step6/1 -> Manual Switch6/1
  Constant4/1 -> Manual Switch6/2
  Manual Switch6/1 -> Subsystem3/1(zref)
  Sum1/1 -> Subsystem1/1(In1)
  Sum/1 -> Subsystem/1(In1)
  Sum2/1 -> Subsystem2/1(In1)
  Subsystem/1(Out1) -> Torque Phi/1
  Subsystem1/1(Out1) -> Torque Theta/1
  Subsystem2/1(Out1) -> Torque Psi/1

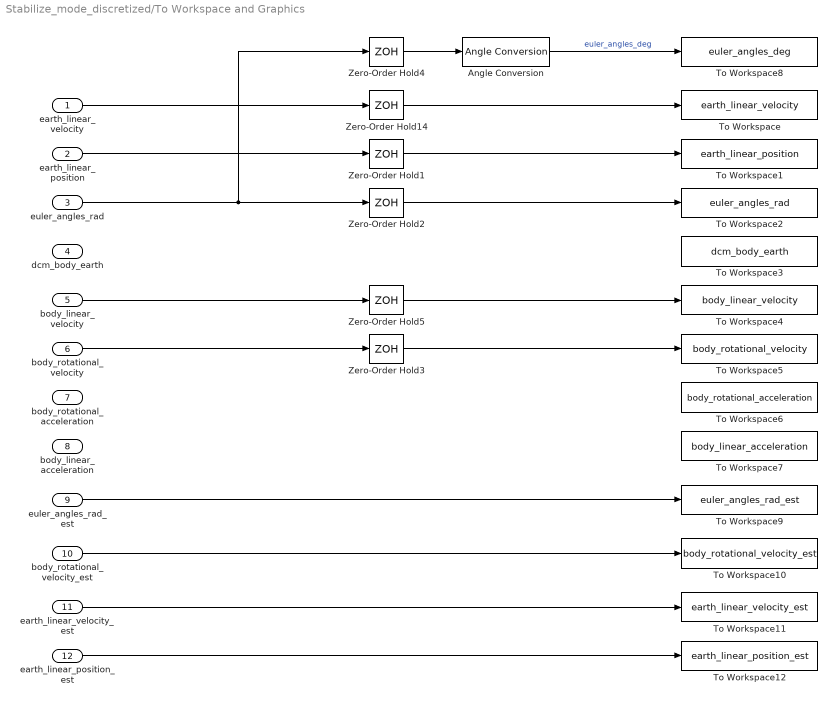
== system Stabilize_mode_discretized/To Workspace and Graphics ==
  earth_linear_velocity : Inport
  earth_linear_position : Inport  Port=2
  euler_angles_rad : Inport  Port=3
  dcm_body_earth : Inport  Port=4
  body_linear_velocity : Inport  Port=5
  body_rotational_velocity : Inport  Port=6
  body_rotational_acceleration : Inport  Port=7
  body_linear_acceleration : Inport  Port=8
  euler_angles_rad_est : Inport  Port=9
  body_rotational_velocity_est : Inport  Port=10
  earth_linear_velocity_est : Inport  Port=11
  earth_linear_position_est : Inport  Port=12
  Angle Conversion : aerolibconvert2/Angle Conversion  IU=rad  OU=deg
  To Workspace : ToWorkspace  VariableName=earth_linear_velocity  SampleTime=-1
  To Workspace1 : ToWorkspace  VariableName=earth_linear_position  SampleTime=-1
  To Workspace10 : ToWorkspace  VariableName=body_rotational_velocity_est  SampleTime=-1
  To Workspace11 : ToWorkspace  VariableName=earth_linear_velocity_est  SampleTime=-1
  To Workspace12 : ToWorkspace  VariableName=earth_linear_position_est  SampleTime=-1
  To Workspace2 : ToWorkspace  VariableName=euler_angles_rad  SampleTime=-1
  To Workspace3 : ToWorkspace  VariableName=dcm_body_earth  SampleTime=-1
  To Workspace4 : ToWorkspace  VariableName=body_linear_velocity  SampleTime=-1
  To Workspace5 : ToWorkspace  VariableName=body_rotational_velocity  SampleTime=-1
  To Workspace6 : ToWorkspace  VariableName=body_rotational_acceleration  SampleTime=-1
  To Workspace7 : ToWorkspace  VariableName=body_linear_acceleration  SampleTime=-1
  To Workspace8 : ToWorkspace  VariableName=euler_angles_deg  SampleTime=-1
  To Workspace9 : ToWorkspace  VariableName=euler_angles_rad_est  SampleTime=-1
  Zero-Order Hold{1..5,14} (6 alike) : ZeroOrderHold  SampleTime=dtzoh
  wires:
  Angle Conversion/1 -> To Workspace8/1  "euler_angles_deg"
  euler_angles_rad/1 -> Zero-Order Hold2/1, Zero-Order Hold4/1
  euler_angles_rad_est/1 -> To Workspace9/1
  earth_linear_position/1 -> Zero-Order Hold1/1
  earth_linear_velocity/1 -> Zero-Order Hold14/1
  earth_linear_position_est/1 -> To Workspace12/1
  earth_linear_velocity_est/1 -> To Workspace11/1
  body_rotational_velocity_est/1 -> To Workspace10/1
  body_rotational_velocity/1 -> Zero-Order Hold3/1
  Zero-Order Hold14/1 -> To Workspace/1
  Zero-Order Hold1/1 -> To Workspace1/1
  Zero-Order Hold2/1 -> To Workspace2/1
  Zero-Order Hold3/1 -> To Workspace5/1
  Zero-Order Hold4/1 -> Angle Conversion/1
  body_linear_velocity/1 -> Zero-Order Hold5/1
  Zero-Order Hold5/1 -> To Workspace4/1

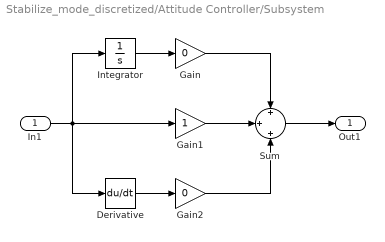
== system Stabilize_mode_discretized/Attitude Controller/Subsystem ==
  In1 : Inport
  Derivative : Derivative
  Gain : Gain  Gain=0
  Gain1 : Gain
  Gain2 : Gain  Gain=0
  Integrator : Integrator
  Sum : Sum  Inputs=+|+|+
  Out1 : Outport
  wires:
  Sum/1 -> Out1/1
  Derivative/1 -> Gain2/1
  Gain2/1 -> Sum/3
  Gain1/1 -> Sum/2
  Gain/1 -> Sum/1
  Integrator/1 -> Gain/1
  In1/1 -> Integrator/1, Derivative/1, Gain1/1

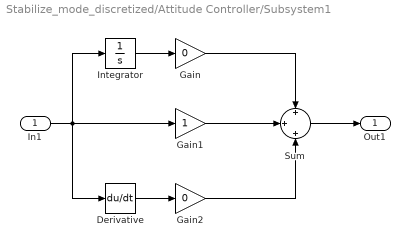
== system Stabilize_mode_discretized/Attitude Controller/Subsystem1 ==
  In1 : Inport
  Derivative : Derivative
  Gain : Gain  Gain=0
  Gain1 : Gain
  Gain2 : Gain  Gain=0
  Integrator : Integrator
  Sum : Sum  Inputs=+|+|+
  Out1 : Outport
  wires:
  Sum/1 -> Out1/1
  Derivative/1 -> Gain2/1
  Gain2/1 -> Sum/3
  Gain1/1 -> Sum/2
  Gain/1 -> Sum/1
  Integrator/1 -> Gain/1
  In1/1 -> Integrator/1, Derivative/1, Gain1/1

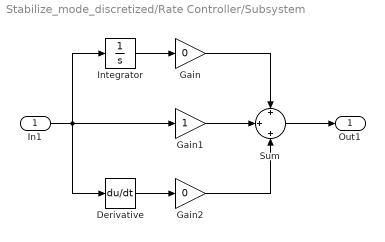
== system Stabilize_mode_discretized/Rate Controller/Subsystem ==
  In1 : Inport
  Derivative : Derivative
  Gain : Gain  Gain=0
  Gain1 : Gain
  Gain2 : Gain  Gain=0
  Integrator : Integrator
  Sum : Sum  Inputs=+|+|+
  Out1 : Outport
  wires:
  Sum/1 -> Out1/1
  Derivative/1 -> Gain2/1
  Gain2/1 -> Sum/3
  Gain1/1 -> Sum/2
  Gain/1 -> Sum/1
  Integrator/1 -> Gain/1
  In1/1 -> Derivative/1, Integrator/1, Gain1/1

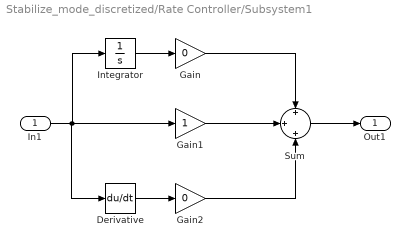
== system Stabilize_mode_discretized/Rate Controller/Subsystem1 ==
  In1 : Inport
  Derivative : Derivative
  Gain : Gain  Gain=0
  Gain1 : Gain
  Gain2 : Gain  Gain=0
  Integrator : Integrator
  Sum : Sum  Inputs=+|+|+
  Out1 : Outport
  wires:
  Sum/1 -> Out1/1
  Derivative/1 -> Gain2/1
  Gain2/1 -> Sum/3
  Gain1/1 -> Sum/2
  Gain/1 -> Sum/1
  Integrator/1 -> Gain/1
  In1/1 -> Gain1/1, Integrator/1, Derivative/1

== system Stabilize_mode_discretized/Rate Controller/Subsystem2 ==
  In1 : Inport
  Derivative : Derivative
  Gain : Gain  Gain=0
  Gain1 : Gain
  Gain2 : Gain
  Integrator : Integrator
  Sum : Sum  Inputs=+|+|+
  Out1 : Outport
  wires:
  Sum/1 -> Out1/1
  Derivative/1 -> Gain2/1
  Gain1/1 -> Sum/2
  Integrator/1 -> Gain/1
  In1/1 -> Integrator/1, Gain1/1

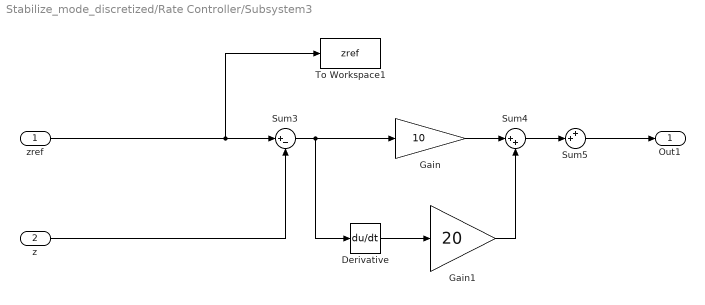
== system Stabilize_mode_discretized/Rate Controller/Subsystem3 ==
  zref : Inport
  z : Inport  Port=2
  Derivative : Derivative
  Gain : Gain  Gain=10
  Gain1 : Gain  Gain=20
  Sum3 : Sum  Inputs=|+-
  Sum4 : Sum  Inputs=|++
  Sum5 : Sum  Inputs=++|
  To Workspace1 : ToWorkspace  VariableName=zref  SampleTime=-1
  Out1 : Outport
  wires:
  z/1 -> Sum3/2
  zref/1 -> To Workspace1/1, Sum3/1
  Derivative/1 -> Gain1/1
  Sum3/1 -> Gain/1, Derivative/1
  Gain1/1 -> Sum4/2
  Sum4/1 -> Sum5/2
  Sum5/1 -> Out1/1
  Gain/1 -> Sum4/1
